simulink model "sol6_LSPB_disturbance"  (R2021b)
settings: Solver=VariableStepAuto  StartTime=0.0  StopTime=1.5  RelTol=1e-3
PreLoadFcn:
  | initModelData
  | trajectoryData
  | controlPID
StartFcn:
  | controlPID
values from neighbouring files (symbols this model uses):
  B = Bm+(Kb*Km/R)    (= 0.0149065789474)    [MyData_for_1_and_2.m]    (also in MyData_for_3_4_and_5.m; MyData_for_5_and_6.m)
  Jm = 5.5e-4    (= 0.00055)    [MyData_for_1_and_2.m]    (also in MyData_for_3_4_and_5.m; MyData_for_5_and_6.m)
  Kd = (R/Km)*((2*Jm*w*zeta)-B)    (= 0.369819047619)    [MyData_for_1_and_2.m]    (also in MyData_for_3_4_and_5.m = 0.2902; MyData_for_5_and_6.m = 0.0513428571429)
  Km = 0.105    [MyData_for_1_and_2.m]    (also in MyData_for_3_4_and_5.m; MyData_for_5_and_6.m)
  Kp = (R/Km)*(Jm*(w^2))    (= 14.3314285714)    [MyData_for_1_and_2.m]    (also in MyData_for_3_4_and_5.m = 9.95238095238; MyData_for_5_and_6.m = 1.59238095238)
  R = 0.76    [MyData_for_1_and_2.m]    (also in MyData_for_3_4_and_5.m; MyData_for_5_and_6.m)
  r = 156    [MyData_for_1_and_2.m]    (also in MyData_for_3_4_and_5.m; MyData_for_5_and_6.m)
undefined symbols (not defined in the file or in its folder): Ki
settings Model: Creator=esdan  LastModifiedBy=munir
settings SolverCC: AlgebraicLoopSolver=TrustRegion
settings DebuggingCC: SFMachineParentedDataDiag=warning

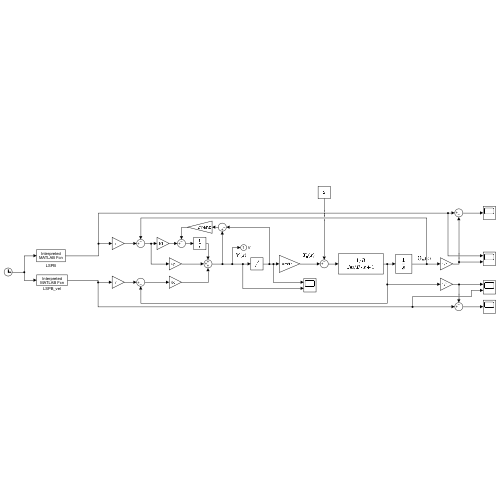
[thumbnail: Simulink's stored preview of the top-level diagram]
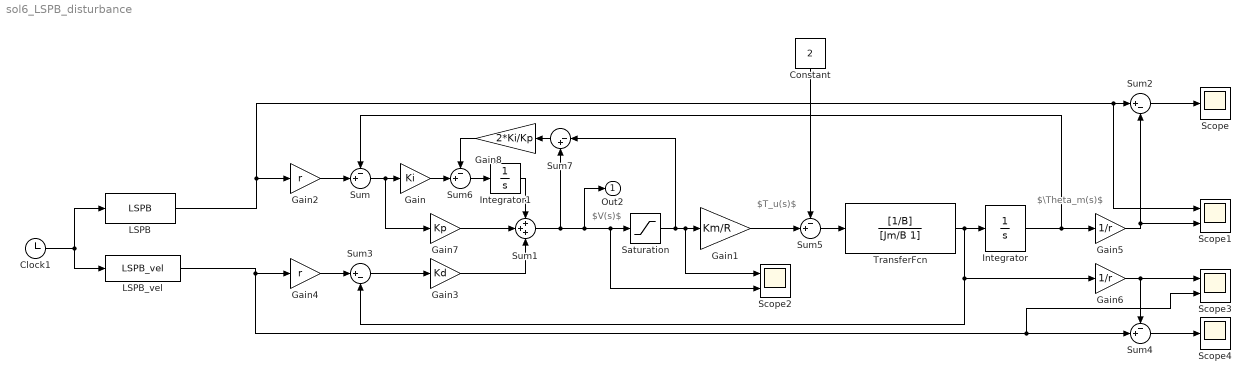
== system sol6_LSPB_disturbance ==
  note: $\Theta_m(s)$
  note: $V(s)$
  note: $T_u(s)$
  Clock1 : Clock
  Constant : Constant  Value=2
  Gain : Gain  Gain=Ki
  Gain1 : Gain  Gain=Km/R
  Gain2 : Gain  Gain=r
  Gain3 : Gain  Gain=Kd
  Gain4 : Gain  Gain=r
  Gain5 : Gain  Gain=1/r
  Gain6 : Gain  Gain=1/r
  Gain7 : Gain  Gain=Kp
  Gain8 : Gain  Gain=2*Ki/Kp
  Integrator : Integrator
  Integrator1 : Integrator
  LSPB : MATLABFcn  MATLABFcn=LSPB
  LSPB_vel : MATLABFcn  MATLABFcn=LSPB_vel
  Saturation : Saturate  UpperLimit=35  LowerLimit=-35
  Scope : Scope
  Scope1 : Scope  NumInputPorts=2
  Scope2 : Scope  NumInputPorts=2
  Scope3 : Scope  NumInputPorts=2
  Scope4 : Scope
  Sum{,4..6} (4 alike) : Sum  Inputs=-+|
  Sum1 : Sum  Inputs=+++
  Sum2 : Sum  Inputs=|+-
  Sum3 : Sum  Inputs=|+-
  Sum7 : Sum  Inputs=|-+
  TransferFcn : TransferFcn  Numerator=[1/B]  Denominator=[Jm/B 1]
  Out2 : Outport  SignalName=V
  wires:
  TransferFcn/1 -> Sum3/2, Gain6/1, Integrator/1
  Saturation/1 -> Sum7/1, Scope2/1, Gain1/1
  Sum/1 -> Gain7/1, Gain/1
  Sum1/1 -> Scope2/2, Saturation/1, Out2/1, Sum7/2
  Gain2/1 -> Sum/2
  LSPB/1 -> Scope1/1, Sum2/1, Gain2/1
  Sum2/1 -> Scope/1
  Sum3/1 -> Gain3/1
  Gain5/1 -> Scope1/2, Sum2/2
  Integrator/1 -> Gain5/1, Sum/1
  LSPB_vel/1 -> Scope3/2, Sum4/2, Gain4/1
  Gain4/1 -> Sum3/1
  Gain6/1 -> Sum4/1, Scope3/1
  Sum5/1 -> TransferFcn/1
  Gain1/1 -> Sum5/2
  Constant/1 -> Sum5/1
  Gain3/1 -> Sum1/3
  Gain7/1 -> Sum1/2
  Gain/1 -> Sum6/2
  Sum7/1 -> Gain8/1
  Gain8/1 -> Sum6/1
  Sum6/1 -> Integrator1/1
  Integrator1/1 -> Sum1/1
  Clock1/1 -> LSPB_vel/1, LSPB/1
  Sum4/1 -> Scope4/1
